simulink model "simulate_FM_Passband"  (R2017a)
settings: Solver=VariableStepAuto  StartTime=0.0  StopTime=inf  RelTol=1e-3
libraries: simulink x1
settings Model: Creator=prust  LastModifiedBy=prust

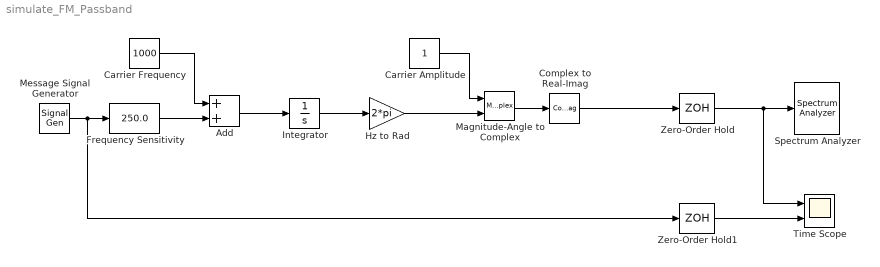
== system simulate_FM_Passband ==
  Add : Sum
  Carrier Amplitude : Constant
  Carrier Frequency : Constant  Value=1000
  Complex to Real-Imag : ComplexToRealImag  Output=Real
  Frequency Sensitivity : simulink/Math Operations/Slider Gain  gain=250.0  low=0  high=500
  Hz to Rad : Gain  Gain=2*pi
  Integrator : Integrator
  Magnitude-Angle to Complex : MagnitudeAngleToComplex
  Message Signal Generator : SignalGenerator  Frequency=50
  Spectrum Analyzer : SpectrumAnalyzer
  Time Scope : Scope  NumInputPorts=2
  Zero-Order Hold : ZeroOrderHold  SampleTime=1/10000
  Zero-Order Hold1 : ZeroOrderHold  SampleTime=1/10000
  wires:
  Message Signal Generator/1 -> Zero-Order Hold1/1, Frequency Sensitivity/1
  Add/1 -> Integrator/1
  Integrator/1 -> Hz to Rad/1
  Carrier Amplitude/1 -> Magnitude-Angle to Complex/1
  Zero-Order Hold/1 -> Spectrum Analyzer/1, Time Scope/1
  Complex to Real-Imag/1 -> Zero-Order Hold/1
  Magnitude-Angle to Complex/1 -> Complex to Real-Imag/1
  Hz to Rad/1 -> Magnitude-Angle to Complex/2
  Zero-Order Hold1/1 -> Time Scope/2
  Frequency Sensitivity/1 -> Add/2
  Carrier Frequency/1 -> Add/1
